simulink model "Arduino_Application"  (Simulink 8.3)
settings: Solver=ode3  SolverMode=SingleTasking  StartTime=0.0  StopTime=inf  RelTol=1e-3
libraries: arduinolib x9
settings Model: Creator=paddockt  LastModifiedBy=paddockt  ExtModeTrigDuration=2
settings DataIOCC: SignalLoggingSaveFormat=Dataset
settings OptimizationCC: OptimizeModelRefInitCode=on  LifeSpan=1
settings DebuggingCC: SolverPrmCheckMsg=none  StateNameClashWarn=none
settings HardwareCC: ProdBitPerInt=16  ProdBitPerPointer=8  ProdIntDivRoundTo=Zero  ProdEndianess=LittleEndian  ProdWordSize=8  ProdHWDeviceType=Atmel->AVR
settings RTWCC: SystemTargetFile=realtime.tlc  GenerateMakefile=off  TemplateMakefile=realtime.tmf  Description=Run on Target Hardware  RTWVerbose=off  ProcessScript=realtime_make_rtw_hook
settings STFCustomTargetCC: TargetLibSuffix=.a  GenerateSampleERTMain=on  ERTCustomFileBanners=on  SupportNonInlinedSFcns=off  SupportVariableSizeSignals=on  MATLABClassNameForMDSCustomization=Simulink.SoftwareTarget.ERTCustomization  GRTInterface=off  SystemTargetFile=realtime.tlc
settings ERTTargetCC: MultiwordLength=2048  GenerateSampleERTMain=on  ParMdlRefBuildCompliant=off  CompOptLevelCompliant=off  ConcurrentExecutionCompliant=off  CombineOutputUpdateFcns=off  ERTFirstTimeCompliant=off  SupportContinuousTime=on  SupportVariableSizeSignals=on  ModelStepFunctionPrototypeControlCompliant=off  CPPClassGenCompliant=off  ExtModeTransport=3  ExtModeMexFile=ext_serial_win32_comm  ExtModeMexArgs=0 1 9600  InlinedParameterPlacement=NonHierarchical  ERTSrcFileBannerTemplate=realtime_code_template.cgt  ERTHdrFileBannerTemplate=realtime_code_template.cgt  ERTDataSrcFileTemplate=realtime_code_template.cgt  ERTDataHdrFileTemplate=realtime_code_template.cgt  ERTCustomFileTemplate=realtime_file_process.tlc  ConvertIfToSwitch=off  SuppressUnreachableDefaultCases=off
settings SettingsController: Description=Run on Hardware Dialog  TargetExtensionPlatform=Arduino Mega 2560
settings MATStruct: Set_host_COM_port=[0.0]  COM_port_number=4  COM_port_baud_rate=115200  Enable_overrun_detection=[0.0]  Digital_output_to_set_on_overrun=13  Extmode_interface_arduino=[0.0]  Analog_input_reference_voltage=[0.0]  Serial0_baud_rate=9600  Serial1_baud_rate=9600  Serial2_baud_rate=9600  Serial3_baud_rate=9600  Local_ip_address=192.168.0.20  Local_mac_address=DE:AD:BE:EF:FE:ED  Wifi_ip_address=192.168.1.20  Wifi_SSID=yourNetwork  Set_Wifi_Encryption=[0.0]  Wifi_WEP_key=D0D0DEADF00DABBADEAFBEADED  Wifi_WEP_key_index=0  Wifi_WPA_password=secretPassword

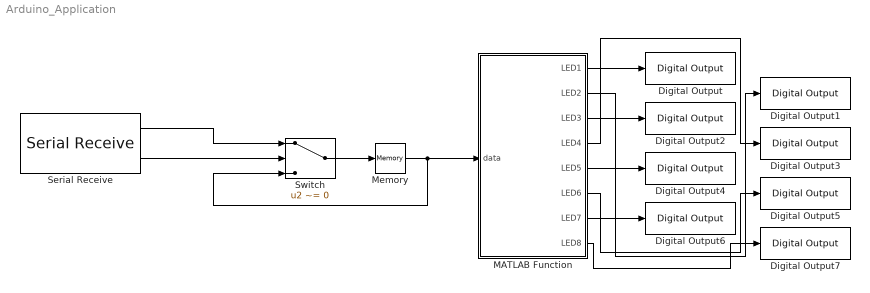
== system Arduino_Application ==
  Digital Output : arduinolib/Digital Output  pinNumber=53
  Digital Output1 : arduinolib/Digital Output  pinNumber=51
  Digital Output2 : arduinolib/Digital Output  pinNumber=49
  Digital Output3 : arduinolib/Digital Output  pinNumber=47
  Digital Output4 : arduinolib/Digital Output  pinNumber=45
  Digital Output5 : arduinolib/Digital Output  pinNumber=43
  Digital Output6 : arduinolib/Digital Output  pinNumber=41
  Digital Output7 : arduinolib/Digital Output  pinNumber=39
  MATLAB Function : MATLAB Function  TreatAsAtomicUnit=on
  Memory : Memory
  Serial Receive : arduinolib/Serial Receive  portNumber=0  showOutStatus=on  sampleTime=1
  Switch : Switch  Criteria=u2 ~= 0
  wires:
  Switch/1 -> Memory/1
  Serial Receive/2 -> Switch/2
  Serial Receive/1 -> Switch/1
  MATLAB Function/1(LED1) -> Digital Output/1
  MATLAB Function/2(LED2) -> Digital Output1/1
  MATLAB Function/3(LED3) -> Digital Output2/1
  MATLAB Function/4(LED4) -> Digital Output3/1
  MATLAB Function/5(LED5) -> Digital Output4/1
  MATLAB Function/6(LED6) -> Digital Output5/1
  MATLAB Function/7(LED7) -> Digital Output6/1
  MATLAB Function/8(LED8) -> Digital Output7/1
  Memory/1 -> Switch/3, MATLAB Function/1(data)

== matlab function MATLAB Function ==
  data: data input double; LED1 output double; LED2 output double; LED3 output double; LED4 output double; LED5 output double; LED6 output double; LED7 output double; LED8 output double
function [LED1, LED2, LED3, LED4, LED5, LED6, LED7, LED8] = fcn(data)
LED1 = mod(data, 2^1);
LED2 = mod(data, 2^2);
LED3 = mod(data, 2^3);
LED4 = mod(data, 2^4);
LED5 = mod(data, 2^5);
LED6 = mod(data, 2^6);
LED7 = mod(data, 2^7);
LED8 = mod(data, 2^8);
